simulink model "NonLinCar"  (Simulink 8.1)
settings: Solver=ode8  StartTime=0.0  StopTime=400  FixedStep=0.001  RelTol=1e-4
settings Model: Creator=rsjoshi1  LastModifiedBy=wyh716  BufferReuse=off
settings SolverCC: EnableConcurrentExecution=on
settings OptimizationCC: BlockReduction=off  BooleanDataType=off  OptimizeBlockIOStorage=off  BufferReuse=off  ExpressionFolding=off  LocalBlockOutputs=off
settings DebuggingCC: SaveWithParameterizedLinksMsg=none  SignalResolutionControl=TryResolveAllWithWarning  SolverPrmCheckMsg=none  MultiTaskDSMMsg=warning  MultiTaskCondExecSysMsg=none  FcnCallInpInsideContextMsg=EnableAllAsWarning
settings HardwareCC: ProdIntDivRoundTo=Zero  ProdEndianess=LittleEndian  ProdHWDeviceType=Generic->32-bit x86 compatible
settings RTWCC: SystemTargetFile=slrt.tlc  TemplateMakefile=slrt_default_tmf  Description=Simulink Real-Time  ProcessScript=slrt_make_rtw_hook  IncludeERTFirstTime=on  RTWCompilerOptimization=On
settings TargetCC: CodeReplacementLibrary=XPC_BLAS  IsPILTarget=off  ParMdlRefBuildCompliant=on  ConcurrentExecutionCompliant=on  MatFileLogging=on  EnableShiftOperators=on  MATLABClassNameForMDSCustomization=xpcAperiodicCustomization
settings CustomProperty: DataType=string  Value=C89/C90 (ANSI)

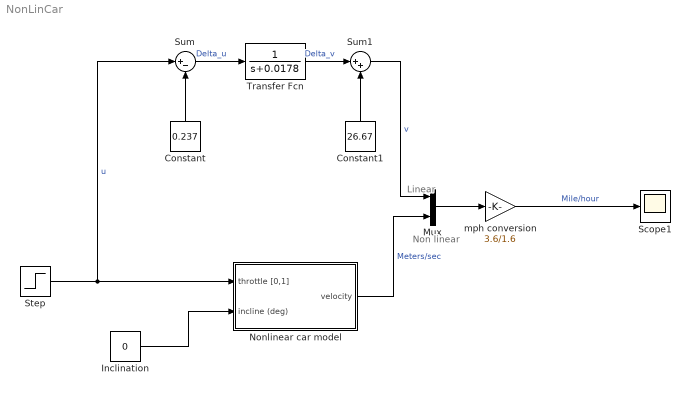
== system NonLinCar ==
  note: Non linear
  note: Linear
  Constant : Constant  Value=0.237
  Constant1 : Constant  Value=26.67
  Inclination : Constant  Value=0
  Mux : Mux  Inputs=2
  Nonlinear car model : Subsystem  mask{ca=1*1500, cf=1*1500/55/55, m=1500}
      mask prompts: ca "acceleration coeff"; cf "friction/aero coeff"; m "mass"
  Scope1 : Scope
      settings: TimeRange=200  YMin=60  YMax=72
  Step : Step  Time=10  Before=0.237  After=0.243  SampleTime=0
  Sum : Sum  Inputs=|+-
  Sum1 : Sum  Inputs=|++
  Transfer Fcn : TransferFcn  Denominator=[1 0.0178]
  mph conversion : Gain  Gain=3.6/1.6  SaturateOnIntegerOverflow=on  OutDataTypeStr=Inherit: Same as input  ParamDataTypeStr=Inherit: Same as input
  wires:
  Step/1 -> Sum/1, Nonlinear car model/1(throttle [0,1])  "u"
  mph conversion/1 -> Scope1/1  "Mile/hour"
  Mux/1 -> mph conversion/1
  Nonlinear car model/1(velocity) -> Mux/2  "Meters/sec"
  Sum/1 -> Transfer Fcn/1  "Delta_u"
  Transfer Fcn/1 -> Sum1/1  "Delta_v"
  Sum1/1 -> Mux/1  "v"
  Constant/1 -> Sum/2
  Constant1/1 -> Sum1/2
  Inclination/1 -> Nonlinear car model/2(incline (deg))

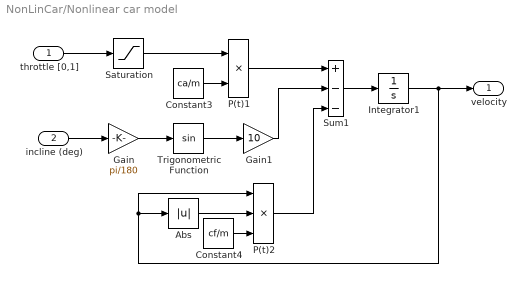
== system NonLinCar/Nonlinear car model ==
  throttle [0,1] : Inport
  incline (deg) : Inport  Port=2
  Abs : Abs  SaturateOnIntegerOverflow=on
  Constant3 : Constant  Value=ca/m
  Constant4 : Constant  Value=cf/m
  Gain : Gain  Gain=pi/180  SaturateOnIntegerOverflow=on  OutDataTypeStr=Inherit: Same as input  ParamDataTypeStr=Inherit: Same as input
  Gain1 : Gain  Gain=10  SaturateOnIntegerOverflow=on  OutDataTypeStr=Inherit: Same as input  ParamDataTypeStr=Inherit: Same as input
  Integrator1 : Integrator  InitialCondition=26.67  UpperSaturationLimit=1  LowerSaturationLimit=0
  P(t)1 : Product  Inputs=**  SaturateOnIntegerOverflow=on  RndMeth=Zero  InputSameDT=on  OutDataTypeStr=Inherit: Same as first input
  P(t)2 : Product  Inputs=***  SaturateOnIntegerOverflow=on  RndMeth=Zero  InputSameDT=on  OutDataTypeStr=Inherit: Same as first input
  Saturation : Saturate  UpperLimit=3  LowerLimit=-1
  Sum1 : Sum  Inputs=+--  SaturateOnIntegerOverflow=on  InputSameDT=on  OutDataTypeStr=Inherit: Same as first input
  Trigonometric Function : Trigonometry
  velocity : Outport
  wires:
  Saturation/1 -> P(t)1/1
  Sum1/1 -> Integrator1/1
  Constant3/1 -> P(t)1/2
  P(t)1/1 -> Sum1/1
  Integrator1/1 -> Abs/1, P(t)2/1, velocity/1
  Constant4/1 -> P(t)2/3
  throttle [0,1]/1 -> Saturation/1
  incline (deg)/1 -> Gain/1
  P(t)2/1 -> Sum1/3
  Gain/1 -> Trigonometric Function/1
  Gain1/1 -> Sum1/2
  Trigonometric Function/1 -> Gain1/1
  Abs/1 -> P(t)2/2
